simulink model "sliding_mode_siso"  (R2017a)
settings: Solver=VariableStepAuto  StartTime=0.0  StopTime=10.0  RelTol=1e-3
undefined symbols (not defined in the file or in its folder): controlfun, plantfun, referencefun, slidingfun, x0, xp0
settings Model: Creator=bruno  LastModifiedBy=bruno

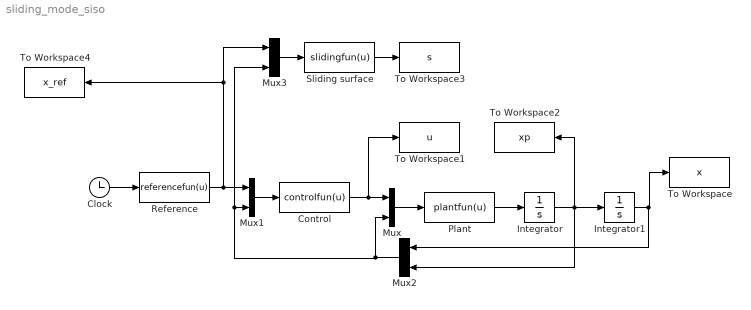
== system sliding_mode_siso ==
  Clock : Clock
  "Control " : MATLABFcn  MATLABFcn=controlfun(u)  OutputSignalType=real
  Integrator : Integrator  InitialCondition=xp0
  Integrator1 : Integrator  InitialCondition=x0
  Mux{,1..3} (4 alike) : Mux  Inputs=2
  Plant : MATLABFcn  MATLABFcn=plantfun(u)  OutputSignalType=real
  Reference : MATLABFcn  MATLABFcn=referencefun(u)  OutputSignalType=real
  Sliding surface : MATLABFcn  MATLABFcn=slidingfun(u)  OutputSignalType=real
  To Workspace : ToWorkspace  VariableName=x  SaveFormat=Timeseries  SampleTime=-1
  To Workspace1 : ToWorkspace  VariableName=u  SaveFormat=Timeseries  SampleTime=-1
  To Workspace2 : ToWorkspace  VariableName=xp  SaveFormat=Timeseries  SampleTime=-1
  To Workspace3 : ToWorkspace  VariableName=s  SaveFormat=Timeseries  SampleTime=-1
  To Workspace4 : ToWorkspace  VariableName=x_ref  SaveFormat=Timeseries  SampleTime=-1
  wires:
  Mux/1 -> Plant/1
  Plant/1 -> Integrator/1
  "Control "/1 -> To Workspace1/1, Mux/1
  Mux1/1 -> "Control "/1
  Clock/1 -> Reference/1
  Reference/1 -> Mux1/1, To Workspace4/1, Mux3/1
  Integrator1/1 -> To Workspace/1, Mux2/1
  Mux2/1 -> Mux3/2, Mux1/2, Mux/2
  Integrator/1 -> Mux2/2, To Workspace2/1, Integrator1/1
  Sliding surface/1 -> To Workspace3/1
  Mux3/1 -> Sliding surface/1
